simulink model "LateralControlDesign"  (R2020b)
settings: Solver=ode15s  StartTime=0.0  StopTime=2.5  RelTol=1e-3
values from neighbouring files (symbols this model uses):
  actuatorDen = [1,   actuatorTimeConstant]    [LateralControl.m]    (also in LongitudinalControl.m)
  actuatorNum = actuatorGain*actuatorTimeConstant    (= 5)    [LateralControl.m]    (also in LongitudinalControl.m)
  ALat = [	-0.256356    	-0.897214    	-125.955 	9.81 ... (first row only)    [LateralControl.m]
  BLat = [	14.7975 ... (first row only)    [LateralControl.m]
  CLat = [1,     0,  0,  0 ... (first row only)    [LateralControl.m]
  DGain = PGain*Td    (= 0.0211)    [LateralControl.m]    (also in LongitudinalControl.m)
  DLat = [0 ... (first row only)    [LateralControl.m]
  InitialConditions = [0 ... (first row only)    [LateralControl.m]    (also in LongitudinalControl.m)
  PGain = 0.211    [LateralControl.m]    (also in LongitudinalControl.m)
  stepCommand = 0    [LateralControl.m]    (also in LongitudinalControl.m = 1)
libraries: slpidlib x1
settings Model: Creator=Antonis Kantounias  LastModifiedBy=Antonis Kantounias

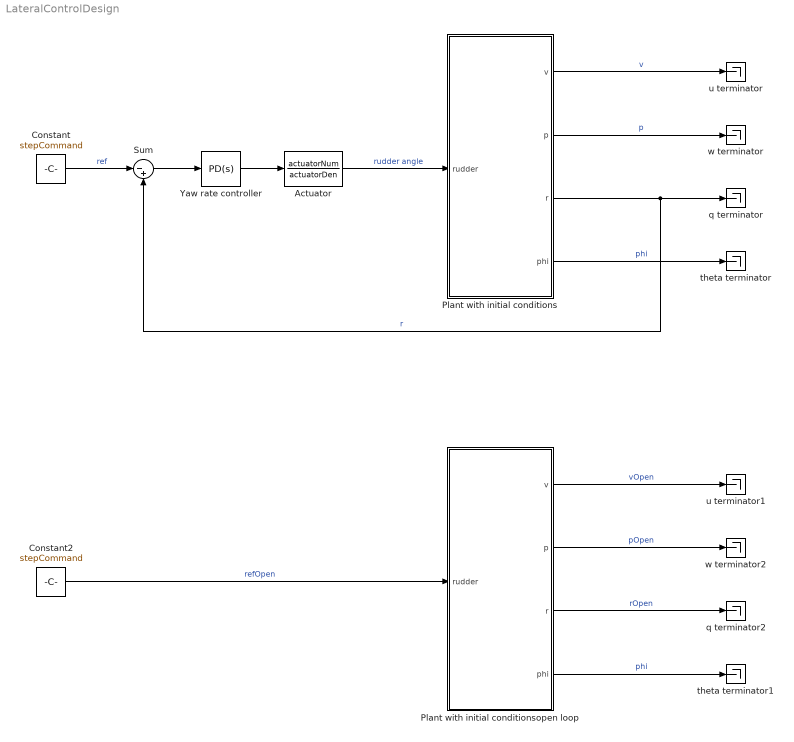
== system LateralControlDesign ==
  Actuator : TransferFcn  Numerator=actuatorNum  Denominator=actuatorDen
  Constant : Constant  Value=stepCommand
  Constant2 : Constant  Value=stepCommand
  Plant with initial conditions : Subsystem
  Plant with initial conditionsopen loop : Subsystem
  Sum : Sum  Inputs=|-+
  Yaw rate controller : slpidlib/PID Controller  Controller=PD  Form=Parallel  TimeDomain=Continuous-time  UseExternalTs=off  SampleTime=-1  IntegratorMethod=Forward Euler  FilterMethod=Forward Euler  ControllerParametersSource=internal  P=PGain  I=1  D=DGain  UseFilter=on  N=50  TunerSelectOption=Transfer Function Based (PID Tuner App)  InitialConditionSource=internal  InitialConditionForIntegrator=0  InitialConditionForFilter=0  DifferentiatorICPrevScaledInput=0  ExternalReset=none  TrackingMode=off  Kt=1  LimitOutput=off  SatLimitsSource=internal  UpperSaturationLimit=inf  LowerSaturationLimit=-inf  LinearizeAsGain=on  AntiWindupMode=none  Kb=1  POutMin=[]  POutMax=[]  IOutMin=[]  IOutMax=[]  DOutMin=[]  DOutMax=[]  NOutMin=[]  NOutMax=[]  SumOutMin=[]  SumOutMax=[]  SaturationOutMin=[]  SaturationOutMax=[]  PParamMin=[]  PParamMax=[]  IParamMin=[]  IParamMax=[]  DParamMin=[]  DParamMax=[]  NParamMin=[]  NParamMax=[]  KbParamMin=[]  KbParamMax=[]  KtParamMin=[]  KtParamMax=[]  KbOutMin=[]  KbOutMax=[]  KtOutMin=[]  KtOutMax=[]  IntegratorOutMin=[]  IntegratorOutMax=[]  FilterOutMin=[]  FilterOutMax=[]  SumI1OutMin=[]  SumI1OutMax=[]  SumI2OutMin=[]  SumI2OutMax=[]  SumI3OutMin=[]  SumI3OutMax=[]  SumI4OutMin=[]  SumI4OutMax=[]  SumDOutMin=[]  SumDOutMax=[]  DifferentiatorOutMin=[]  DifferentiatorOutMax=[]  FilterDiffOutCoefMin=[]  FilterDiffOutCoefMax=[]  ReciprocalOutMin=[]  ReciprocalOutMax=[]  SumDenOutMin=[]  SumDenOutMax=[]  SumNumOutMin=[]  SumNumOutMax=[]  DivideOutMin=[]  DivideOutMax=[]  UdiffTsProdOutMin=[]  UdiffTsProdOutMax=[]  NTsProdOutMin=[]  NTsProdOutMax=[]  UintegralTsProdOutMin=[]  UintegralTsProdOutMax=[]  UngainTsProdOutMin=[]  UngainTsProdOutMax=[]  IntegratorContinuousStateAttributes=''  IntegratorStateMustResolveToSignalObject=off  IntegratorRTWStateStorageClass=Auto  FilterContinuousStateAttributes=''  FilterStateMustResolveToSignalObject=off  FilterRTWStateStorageClass=Auto  ParallelPVariant=InternalParameters  IdealPVariant=Disabled  IVariant=Disabled  DVariant=InternalParameters  IntegratorVariant=Disabled  SatVariant=Disabled  AWVariant=Disabled  PCopyVariant=Disabled  TRVariant=Disabled  FdbkBlocksVariant=Forward  IdealPFdbkVariant=Disabled  SatFdbkVariant=Disabled  DerivativeFilterVariant=ContFilter  NVariant=InternalParameters  NCopyVariant=Disabled  FilterICVariant=InternalICsFilter  IntegratorICVariant=Disabled  ExternalResetVariant=Disabled  TRSumVariant=Passthrough  SumFdbkVariant=Disabled  SumVariant=Sum_PD  TsampFilterVariant=InternalTs  TsampNgainVariant=Passthrough  TsampIntegralVariant=Disabled_SignalSpec  ExternalSaturationOutDataTypeStr=Inherit: Same as second input
  q terminator : Terminator
  q terminator2 : Terminator
  theta terminator : Terminator
  theta terminator1 : Terminator
  u terminator : Terminator
  u terminator1 : Terminator
  w terminator : Terminator
  w terminator2 : Terminator
  wires:
  Plant with initial conditions/3(r) -> q terminator/1, Sum/2  "r"
  Plant with initial conditions/1(v) -> u terminator/1  "v"
  Plant with initial conditions/2(p) -> w terminator/1  "p"
  Plant with initial conditions/4(phi) -> theta terminator/1  "phi"
  Constant/1 -> Sum/1  "ref"
  Sum/1 -> Yaw rate controller/1
  Yaw rate controller/1 -> Actuator/1
  Actuator/1 -> Plant with initial conditions/1(rudder)  "rudder angle"
  Constant2/1 -> Plant with initial conditionsopen loop/1(rudder)  "refOpen"
  Plant with initial conditionsopen loop/4(phi) -> theta terminator1/1  "phi"
  Plant with initial conditionsopen loop/1(v) -> u terminator1/1  "vOpen"
  Plant with initial conditionsopen loop/2(p) -> w terminator2/1  "pOpen"
  Plant with initial conditionsopen loop/3(r) -> q terminator2/1  "rOpen"

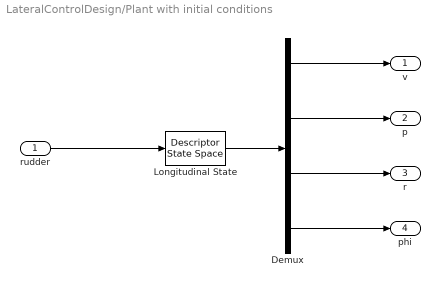
== system LateralControlDesign/Plant with initial conditions ==
  rudder : Inport
  Demux : Demux
  "Longitudinal State " : DescriptorStateSpace  E=ELat  A=ALat  B=BLat  C=CLat  D=DLat  InitialCondition=InitialConditions  ContinuousStateAttributes='LateralSystem'
  v : Outport
  p : Outport  Port=2
  r : Outport  Port=3
  phi : Outport  Port=4
  wires:
  "Longitudinal State "/1 -> Demux/1
  Demux/4 -> phi/1
  Demux/1 -> v/1
  Demux/3 -> r/1
  Demux/2 -> p/1
  rudder/1 -> "Longitudinal State "/1

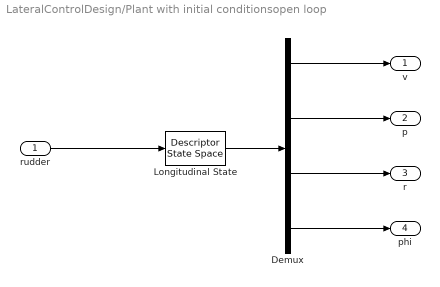
== system LateralControlDesign/Plant with initial conditionsopen loop ==
  rudder : Inport
  Demux : Demux
  "Longitudinal State " : DescriptorStateSpace  E=ELat  A=ALat  B=BLat  C=CLat  D=DLat  InitialCondition=InitialConditions  ContinuousStateAttributes='LongitudinalSystem'
  v : Outport
  p : Outport  Port=2
  r : Outport  Port=3
  phi : Outport  Port=4
  wires:
  rudder/1 -> "Longitudinal State "/1
  Demux/2 -> p/1
  Demux/3 -> r/1
  Demux/1 -> v/1
  Demux/4 -> phi/1
  "Longitudinal State "/1 -> Demux/1
